simulink model "f4_variable_load"  (R2019b)
settings: Solver=VariableStepAuto  StartTime=0.0  StopTime=20  RelTol=1e-3
libraries: powerlib x28
settings Model: Creator=MAHMUD  LastModifiedBy=MAHMUD
settings DataIOCC: ReturnWorkspaceOutputs=off
settings DebuggingCC: ArithmeticOperatorsInVariantConditions=warning
settings SFSimCC: SimUseLocalCustomCode=off  CustomCodeUndefinedFunction=UseInterfaceOnly
settings RTWCC: RTWUseLocalCustomCode=off

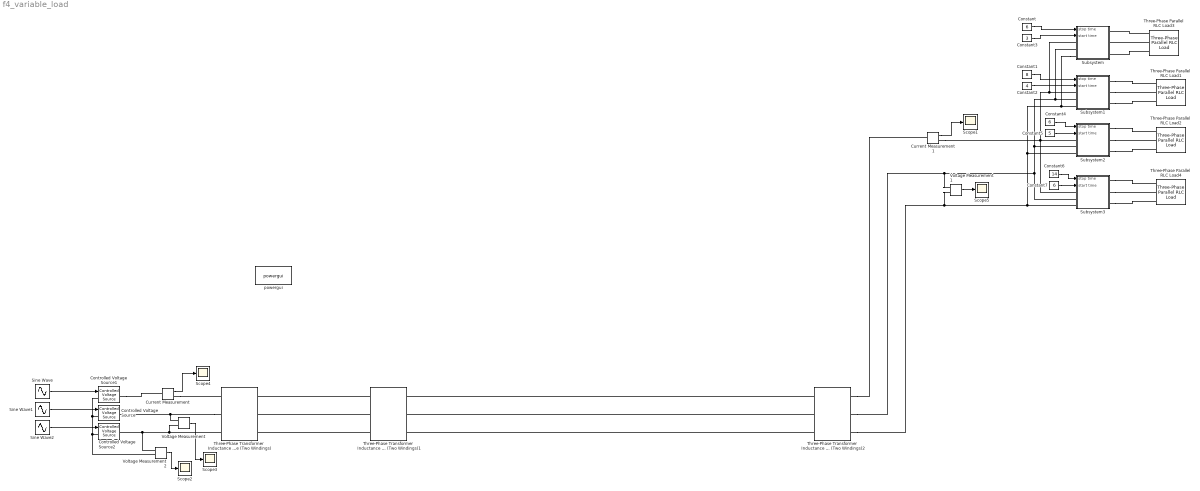
== system f4_variable_load ==
  Constant : Constant  Value=6
  Constant1 : Constant  Value=8
  Constant2 : Constant  Value=4
  Constant3 : Constant  Value=3
  Constant4 : Constant  Value=6
  Constant5 : Constant  Value=5
  Constant6 : Constant  Value=14
  Constant7 : Constant  Value=6
  Controlled Voltage Source : powerlib/Electrical Sources/Controlled Voltage Source  Initialize=on  Source_Type=AC  Amplitude=0  Phase=0  Frequency=0  Measurements=None
      settings: SourceProductName=Simscape Electrical
  Controlled Voltage Source1 : powerlib/Electrical Sources/Controlled Voltage Source  Initialize=on  Source_Type=AC  Amplitude=0  Phase=0  Frequency=0  Measurements=None
      settings: SourceProductName=Simscape Electrical
  Controlled Voltage Source2 : powerlib/Electrical Sources/Controlled Voltage Source  Initialize=on  Source_Type=AC  Amplitude=0  Phase=0  Frequency=0  Measurements=None
      settings: SourceProductName=Simscape Electrical
  Current Measurement : powerlib/Measurements/Current Measurement  PhasorSimulation=off  OutputType=Complex  PSBequivalent=0
      settings: SourceProductName=Simscape Electrical
  Current Measurement1 : powerlib/Measurements/Current Measurement  PhasorSimulation=off  OutputType=Complex  PSBequivalent=0
      settings: SourceProductName=Simscape Electrical
  Scope{1..5} (5 alike) : Scope
  Sine Wave : Sin  Amplitude=11500  Frequency=50*2*pi  SampleTime=0
  Sine Wave1 : Sin  Amplitude=11500  Frequency=50*2*pi  Phase=pi*2/3  SampleTime=0
  Sine Wave2 : Sin  Amplitude=11500  Frequency=50*2*pi  Phase=4*pi/3  SampleTime=0
  Subsystem : Subsystem
  Subsystem1 : Subsystem
  Subsystem2 : Subsystem
  Subsystem3 : Subsystem
  Three-Phase Parallel RLC Load1 : powerlib/Elements/Three-Phase Parallel RLC Load  LConnTagsString=A|B|C  Configuration=Y (grounded)  NominalVoltage=220  Vabc=[1e3 1e3 1e3]  Vabcp=[1e3 1e3 1e3]  NominalFrequency=50  UnbalancedPower=off  ActivePower=1.5e3  InductivePower=100  CapacitivePower=100  Pabc=[10e3 9e3 11e3]  QLabc=[100 90 110]  QCabc=[100 90 110]  Pabcp=[10e3 9e3 11e3]  QLabcp=[100 90 110]  QCabcp=[100 90 110]  Measurements=None  LoadType=constant Z
      settings: SourceProductName=Simscape Electrical
  Three-Phase Parallel RLC Load2 : powerlib/Elements/Three-Phase Parallel RLC Load  LConnTagsString=A|B|C  Configuration=Y (grounded)  NominalVoltage=220  Vabc=[1e3 1e3 1e3]  Vabcp=[1e3 1e3 1e3]  NominalFrequency=50  UnbalancedPower=off  ActivePower=1e3  InductivePower=100  CapacitivePower=100  Pabc=[10e3 9e3 11e3]  QLabc=[100 90 110]  QCabc=[100 90 110]  Pabcp=[10e3 9e3 11e3]  QLabcp=[100 90 110]  QCabcp=[100 90 110]  Measurements=None  LoadType=constant Z
      settings: SourceProductName=Simscape Electrical
  Three-Phase Parallel RLC Load3 : powerlib/Elements/Three-Phase Parallel RLC Load  LConnTagsString=A|B|C  Configuration=Y (grounded)  NominalVoltage=220  Vabc=[1e3 1e3 1e3]  Vabcp=[1e3 1e3 1e3]  NominalFrequency=50  UnbalancedPower=off  ActivePower=4e3  InductivePower=100  CapacitivePower=100  Pabc=[10e3 9e3 11e3]  QLabc=[100 90 110]  QCabc=[100 90 110]  Pabcp=[10e3 9e3 11e3]  QLabcp=[100 90 110]  QCabcp=[100 90 110]  Measurements=None  LoadType=constant Z
      settings: SourceProductName=Simscape Electrical
  Three-Phase Parallel RLC Load4 : powerlib/Elements/Three-Phase Parallel RLC Load  LConnTagsString=A|B|C  Configuration=Y (grounded)  NominalVoltage=220  Vabc=[1e3 1e3 1e3]  Vabcp=[1e3 1e3 1e3]  NominalFrequency=50  UnbalancedPower=off  ActivePower=12e3  InductivePower=100  CapacitivePower=100  Pabc=[10e3 9e3 11e3]  QLabc=[100 90 110]  QCabc=[100 90 110]  Pabcp=[10e3 9e3 11e3]  QLabcp=[100 90 110]  QCabcp=[100 90 110]  Measurements=None  LoadType=constant Z
      settings: SourceProductName=Simscape Electrical
  Three-Phase Transformer Inductance Matrix Type (Two Windings) : powerlib/Elements/Three-Phase Transformer Inductance Matrix Type (Two Windings)  CoreType=Three-limb or five-limb core  Winding1Connection=Yg  Winding2Connection=Yg  AutoTransformer=off  Measurements=None  NominalPower=[100e3, 50]  VLLnom=[25000, 130000]  WindingResistances=[0.01, 0.01]  NoLoadIexcPos=2  NoLoadPlossPos=1000  ShortCircuitReactancePos=0.06  ShortCircuitReactancePosAuto=0.06  NoLoadIexcZero=100  NoLoadPlossZero=1500  ShortCircuitReactanceZero=0.03  ShortCircuitReactanceZeroAuto=0.03
      settings: SourceProductName=Simscape Electrical  SourceProductBaseCode=PS
  Three-Phase Transformer Inductance Matrix Type (Two Windings)1 : powerlib/Elements/Three-Phase Transformer Inductance Matrix Type (Two Windings)  CoreType=Three-limb or five-limb core  Winding1Connection=Yg  Winding2Connection=Yg  AutoTransformer=off  Measurements=None  NominalPower=[100e3, 50]  VLLnom=[130000, 11000]  WindingResistances=[0.01, 0.01]  NoLoadIexcPos=2  NoLoadPlossPos=1000  ShortCircuitReactancePos=0.06  ShortCircuitReactancePosAuto=0.06  NoLoadIexcZero=100  NoLoadPlossZero=1500  ShortCircuitReactanceZero=0.03  ShortCircuitReactanceZeroAuto=0.03
      settings: SourceProductName=Simscape Electrical  SourceProductBaseCode=PS
  Three-Phase Transformer Inductance Matrix Type (Two Windings)2 : powerlib/Elements/Three-Phase Transformer Inductance Matrix Type (Two Windings)  CoreType=Three-limb or five-limb core  Winding1Connection=Yg  Winding2Connection=Yg  AutoTransformer=off  Measurements=None  NominalPower=[100e3, 50]  VLLnom=[11000, 381]  WindingResistances=[0.01, 0.01]  NoLoadIexcPos=2  NoLoadPlossPos=1000  ShortCircuitReactancePos=0.06  ShortCircuitReactancePosAuto=0.06  NoLoadIexcZero=100  NoLoadPlossZero=1500  ShortCircuitReactanceZero=0.03  ShortCircuitReactanceZeroAuto=0.03
      settings: SourceProductName=Simscape Electrical  SourceProductBaseCode=PS
  Voltage Measurement : powerlib/Measurements/Voltage Measurement  PhasorSimulation=off  OutputType=Complex  PSBequivalent=0
      settings: SourceProductName=Simscape Electrical
  Voltage Measurement1 : powerlib/Measurements/Voltage Measurement  PhasorSimulation=off  OutputType=Complex  PSBequivalent=0
      settings: SourceProductName=Simscape Electrical
  Voltage Measurement2 : powerlib/Measurements/Voltage Measurement  PhasorSimulation=off  OutputType=Complex  PSBequivalent=0
      settings: SourceProductName=Simscape Electrical
  powergui : powerlib/powergui  Priority=1  SimulationMode=Continuous  SampleTime=50e-6  frequency=60  Iterations=50  frequencyindice=50  Pbase=100e6  ErrMax=1e-4  UnitsV=kV  UnitsW=MW  buscounter=0  FunctionMessages=off  echomessages=off  EnableUseOfTLC=off  CurrentSourceSwitches=off  DisableSnubberDevices=off  DisableRonSwitches=off  DisableVfSwitches=off  DisplayEquations=off  AutomaticDiscreteSolvers=off  SolverType=Tustin/Backward Euler (TBE)  Interpol=off  ExternalGateDelay=off  methode=off  Ts=100  x0status=blocks  SPID=on  SwTol=0  HookPort=off  NonlinearTolerance=1e-4  nMaxIteration=100  ContinueOnMaxIteration=off  RestoreLinks=warning  ResistiveCurrentMeasurement=off  Frange=[0:2:500]  Ylog=off  Xlog=on  ShowGrid=off  save=off  variable=ZData  structure=0  ZoomFFT=off  StartTime=0.0  cycles=1  DisplayStyle=1  fundamental=60  FreqAxis=off  MaxFrequency=1000  frequencyindicesteady=1  RmsSteady=1  display=off
      settings: SourceProductName=Simscape Electrical
  wires:
  Voltage Measurement2/1 -> Scope2/1
  Constant5/1 -> Subsystem2/2(start time)
  Current Measurement/1 -> Scope4/1
  Constant1/1 -> Subsystem1/1(stop time)
  Constant6/1 -> Subsystem3/1(stop time)
  Sine Wave1/1 -> Controlled Voltage Source/1
  Sine Wave2/1 -> Controlled Voltage Source2/1
  Voltage Measurement1/1 -> Scope5/1
  Voltage Measurement/1 -> Scope3/1
  Constant7/1 -> Subsystem3/2(start time)
  Constant3/1 -> Subsystem/2(start time)
  Constant2/1 -> Subsystem1/2(start time)
  Constant/1 -> Subsystem/1(stop time)
  Constant4/1 -> Subsystem2/1(stop time)
  Sine Wave/1 -> Controlled Voltage Source1/1
  Current Measurement1/1 -> Scope1/1
  connections:
  Subsystem/LConn3 -- Subsystem1/LConn3 -- Subsystem2/LConn3 -- Voltage Measurement1/LConn2 -- Three-Phase Transformer Inductance Matrix Type (Two Windings)2/RConn3 -- Subsystem3/LConn3
  Controlled Voltage Source2/LConn1 -- Voltage Measurement2/LConn2 -- Controlled Voltage Source1/LConn1 -- Controlled Voltage Source/LConn1
  Three-Phase Transformer Inductance Matrix Type (Two Windings)/LConn2 -- Controlled Voltage Source/RConn1 -- Voltage Measurement/LConn1
  Three-Phase Transformer Inductance Matrix Type (Two Windings)2/RConn2 -- Voltage Measurement1/LConn1 -- Subsystem3/LConn2 -- Subsystem/LConn2 -- Subsystem1/LConn2 -- Subsystem2/LConn2
  Controlled Voltage Source2/RConn1 -- Voltage Measurement2/LConn1 -- Three-Phase Transformer Inductance Matrix Type (Two Windings)/LConn3 -- Voltage Measurement/LConn2
  Subsystem3/LConn1 -- Subsystem/LConn1 -- Subsystem1/LConn1 -- Subsystem2/LConn1 -- Current Measurement1/RConn1
  Three-Phase Transformer Inductance Matrix Type (Two Windings)2/LConn1 -- Three-Phase Transformer Inductance Matrix Type (Two Windings)1/RConn1
  Three-Phase Parallel RLC Load3/LConn2 -- Subsystem/RConn2
  Subsystem1/RConn2 -- Three-Phase Parallel RLC Load1/LConn2
  Three-Phase Parallel RLC Load3/LConn3 -- Subsystem/RConn3
  Three-Phase Transformer Inductance Matrix Type (Two Windings)2/LConn2 -- Three-Phase Transformer Inductance Matrix Type (Two Windings)1/RConn2
  Current Measurement/RConn1 -- Three-Phase Transformer Inductance Matrix Type (Two Windings)/LConn1
  Three-Phase Parallel RLC Load3/LConn1 -- Subsystem/RConn1
  Subsystem3/RConn3 -- Three-Phase Parallel RLC Load4/LConn3
  Controlled Voltage Source1/RConn1 -- Current Measurement/LConn1
  Three-Phase Transformer Inductance Matrix Type (Two Windings)2/LConn3 -- Three-Phase Transformer Inductance Matrix Type (Two Windings)1/RConn3
  Subsystem1/RConn3 -- Three-Phase Parallel RLC Load1/LConn3
  Three-Phase Transformer Inductance Matrix Type (Two Windings)1/LConn3 -- Three-Phase Transformer Inductance Matrix Type (Two Windings)/RConn3
  Three-Phase Transformer Inductance Matrix Type (Two Windings)2/RConn1 -- Current Measurement1/LConn1
  Subsystem3/RConn1 -- Three-Phase Parallel RLC Load4/LConn1
  Three-Phase Transformer Inductance Matrix Type (Two Windings)1/LConn2 -- Three-Phase Transformer Inductance Matrix Type (Two Windings)/RConn2
  Subsystem3/RConn2 -- Three-Phase Parallel RLC Load4/LConn2
  Subsystem1/RConn1 -- Three-Phase Parallel RLC Load1/LConn1
  Subsystem2/RConn1 -- Three-Phase Parallel RLC Load2/LConn1
  Three-Phase Transformer Inductance Matrix Type (Two Windings)1/LConn1 -- Three-Phase Transformer Inductance Matrix Type (Two Windings)/RConn1
  Subsystem2/RConn2 -- Three-Phase Parallel RLC Load2/LConn2
  Subsystem2/RConn3 -- Three-Phase Parallel RLC Load2/LConn3

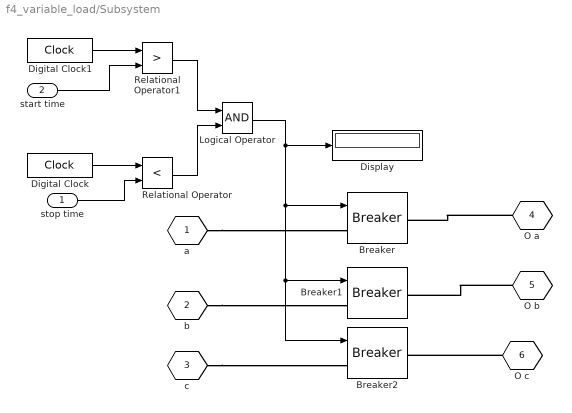
== system f4_variable_load/Subsystem ==
  stop time : Inport
  start time : Inport  Port=2
  Breaker : powerlib/Elements/Breaker  InitialState=0  SwitchingTimes="[1/60  5/60]"  External=on  BreakerResistance=0.01  SnubberResistance=1e6  SnubberCapacitance=inf  Measurements=None  MoreParameters=on  NoBreakLoop=off
      settings: SourceProductName=Simscape Electrical
  Breaker1 : powerlib/Elements/Breaker  InitialState=0  SwitchingTimes="[1/60  5/60]"  External=on  BreakerResistance=0.01  SnubberResistance=1e6  SnubberCapacitance=inf  Measurements=None  MoreParameters=on  NoBreakLoop=off
      settings: SourceProductName=Simscape Electrical
  Breaker2 : powerlib/Elements/Breaker  InitialState=0  SwitchingTimes="[1/60  5/60]"  External=on  BreakerResistance=0.01  SnubberResistance=1e6  SnubberCapacitance=inf  Measurements=None  MoreParameters=on  NoBreakLoop=off
      settings: SourceProductName=Simscape Electrical
  Digital Clock : DigitalClock
  Digital Clock1 : DigitalClock
  Display : Display
  Logical Operator : Logic  AllPortsSameDT=off  OutDataTypeStr=boolean
  Relational Operator : RelationalOperator  Operator=<  OutDataTypeStr=boolean  RndMeth=Simplest
  Relational Operator1 : RelationalOperator  Operator=>  OutDataTypeStr=boolean  RndMeth=Simplest
  a : PMIOPort  Tag=PMCPort  Side=Left
  b : PMIOPort  Tag=PMCPort  Port=2  Side=Left
  c : PMIOPort  Tag=PMCPort  Port=3  Side=Left
  "O a " : PMIOPort  Tag=PMCPort  Port=4  Side=Right
  O b : PMIOPort  Tag=PMCPort  Port=5  Side=Right
  O c : PMIOPort  Tag=PMCPort  Port=6  Side=Right
  wires:
  Logical Operator/1 -> Breaker/1, Breaker2/1, Breaker1/1, Display/1
  Digital Clock/1 -> Relational Operator/1
  stop time/1 -> Relational Operator/2
  Digital Clock1/1 -> Relational Operator1/1
  start time/1 -> Relational Operator1/2
  Relational Operator1/1 -> Logical Operator/1
  Relational Operator/1 -> Logical Operator/2
  connections:
  O c/RConn1 -- Breaker2/RConn1
  b/RConn1 -- Breaker1/LConn1
  O b/RConn1 -- Breaker1/RConn1
  c/RConn1 -- Breaker2/LConn1
  "O a "/RConn1 -- Breaker/RConn1
  a/RConn1 -- Breaker/LConn1

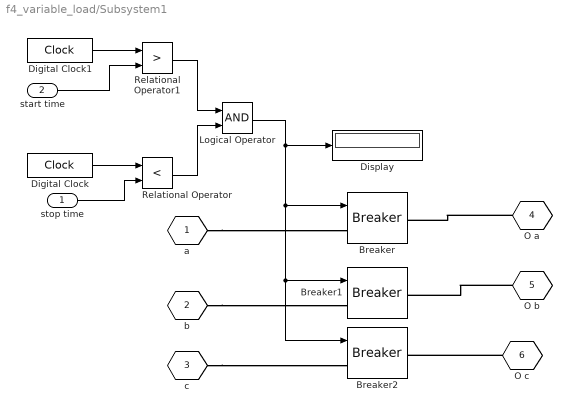
== system f4_variable_load/Subsystem1 ==
  stop time : Inport
  start time : Inport  Port=2
  Breaker : powerlib/Elements/Breaker  InitialState=0  SwitchingTimes="[1/60  5/60]"  External=on  BreakerResistance=0.01  SnubberResistance=1e6  SnubberCapacitance=inf  Measurements=None  MoreParameters=on  NoBreakLoop=off
      settings: SourceProductName=Simscape Electrical
  Breaker1 : powerlib/Elements/Breaker  InitialState=0  SwitchingTimes="[1/60  5/60]"  External=on  BreakerResistance=0.01  SnubberResistance=1e6  SnubberCapacitance=inf  Measurements=None  MoreParameters=on  NoBreakLoop=off
      settings: SourceProductName=Simscape Electrical
  Breaker2 : powerlib/Elements/Breaker  InitialState=0  SwitchingTimes="[1/60  5/60]"  External=on  BreakerResistance=0.01  SnubberResistance=1e6  SnubberCapacitance=inf  Measurements=None  MoreParameters=on  NoBreakLoop=off
      settings: SourceProductName=Simscape Electrical
  Digital Clock : DigitalClock
  Digital Clock1 : DigitalClock
  Display : Display
  Logical Operator : Logic  AllPortsSameDT=off  OutDataTypeStr=boolean
  Relational Operator : RelationalOperator  Operator=<  OutDataTypeStr=boolean  RndMeth=Simplest
  Relational Operator1 : RelationalOperator  Operator=>  OutDataTypeStr=boolean  RndMeth=Simplest
  a : PMIOPort  Tag=PMCPort  Side=Left
  b : PMIOPort  Tag=PMCPort  Port=2  Side=Left
  c : PMIOPort  Tag=PMCPort  Port=3  Side=Left
  "O a " : PMIOPort  Tag=PMCPort  Port=4  Side=Right
  O b : PMIOPort  Tag=PMCPort  Port=5  Side=Right
  O c : PMIOPort  Tag=PMCPort  Port=6  Side=Right
  wires:
  Relational Operator/1 -> Logical Operator/2
  Relational Operator1/1 -> Logical Operator/1
  start time/1 -> Relational Operator1/2
  Digital Clock1/1 -> Relational Operator1/1
  stop time/1 -> Relational Operator/2
  Digital Clock/1 -> Relational Operator/1
  Logical Operator/1 -> Display/1, Breaker1/1, Breaker2/1, Breaker/1
  connections:
  a/RConn1 -- Breaker/LConn1
  "O a "/RConn1 -- Breaker/RConn1
  c/RConn1 -- Breaker2/LConn1
  O b/RConn1 -- Breaker1/RConn1
  b/RConn1 -- Breaker1/LConn1
  O c/RConn1 -- Breaker2/RConn1

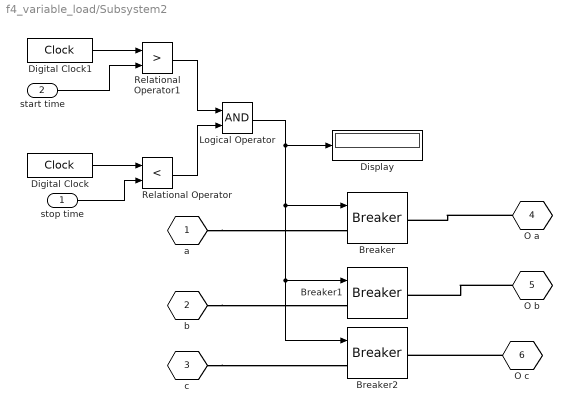
== system f4_variable_load/Subsystem2 ==
  stop time : Inport
  start time : Inport  Port=2
  Breaker : powerlib/Elements/Breaker  InitialState=0  SwitchingTimes="[1/60  5/60]"  External=on  BreakerResistance=0.01  SnubberResistance=1e6  SnubberCapacitance=inf  Measurements=None  MoreParameters=on  NoBreakLoop=off
      settings: SourceProductName=Simscape Electrical
  Breaker1 : powerlib/Elements/Breaker  InitialState=0  SwitchingTimes="[1/60  5/60]"  External=on  BreakerResistance=0.01  SnubberResistance=1e6  SnubberCapacitance=inf  Measurements=None  MoreParameters=on  NoBreakLoop=off
      settings: SourceProductName=Simscape Electrical
  Breaker2 : powerlib/Elements/Breaker  InitialState=0  SwitchingTimes="[1/60  5/60]"  External=on  BreakerResistance=0.01  SnubberResistance=1e6  SnubberCapacitance=inf  Measurements=None  MoreParameters=on  NoBreakLoop=off
      settings: SourceProductName=Simscape Electrical
  Digital Clock : DigitalClock
  Digital Clock1 : DigitalClock
  Display : Display
  Logical Operator : Logic  AllPortsSameDT=off  OutDataTypeStr=boolean
  Relational Operator : RelationalOperator  Operator=<  OutDataTypeStr=boolean  RndMeth=Simplest
  Relational Operator1 : RelationalOperator  Operator=>  OutDataTypeStr=boolean  RndMeth=Simplest
  a : PMIOPort  Tag=PMCPort  Side=Left
  b : PMIOPort  Tag=PMCPort  Port=2  Side=Left
  c : PMIOPort  Tag=PMCPort  Port=3  Side=Left
  "O a " : PMIOPort  Tag=PMCPort  Port=4  Side=Right
  O b : PMIOPort  Tag=PMCPort  Port=5  Side=Right
  O c : PMIOPort  Tag=PMCPort  Port=6  Side=Right
  wires:
  Logical Operator/1 -> Breaker/1, Breaker2/1, Breaker1/1, Display/1
  Digital Clock/1 -> Relational Operator/1
  stop time/1 -> Relational Operator/2
  Digital Clock1/1 -> Relational Operator1/1
  start time/1 -> Relational Operator1/2
  Relational Operator1/1 -> Logical Operator/1
  Relational Operator/1 -> Logical Operator/2
  connections:
  O c/RConn1 -- Breaker2/RConn1
  b/RConn1 -- Breaker1/LConn1
  O b/RConn1 -- Breaker1/RConn1
  c/RConn1 -- Breaker2/LConn1
  "O a "/RConn1 -- Breaker/RConn1
  a/RConn1 -- Breaker/LConn1

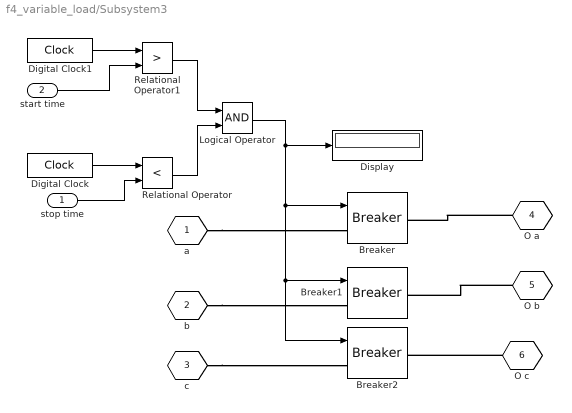
== system f4_variable_load/Subsystem3 ==
  stop time : Inport
  start time : Inport  Port=2
  Breaker : powerlib/Elements/Breaker  InitialState=0  SwitchingTimes="[1/60  5/60]"  External=on  BreakerResistance=0.01  SnubberResistance=1e6  SnubberCapacitance=inf  Measurements=None  MoreParameters=on  NoBreakLoop=off
      settings: SourceProductName=Simscape Electrical
  Breaker1 : powerlib/Elements/Breaker  InitialState=0  SwitchingTimes="[1/60  5/60]"  External=on  BreakerResistance=0.01  SnubberResistance=1e6  SnubberCapacitance=inf  Measurements=None  MoreParameters=on  NoBreakLoop=off
      settings: SourceProductName=Simscape Electrical
  Breaker2 : powerlib/Elements/Breaker  InitialState=0  SwitchingTimes="[1/60  5/60]"  External=on  BreakerResistance=0.01  SnubberResistance=1e6  SnubberCapacitance=inf  Measurements=None  MoreParameters=on  NoBreakLoop=off
      settings: SourceProductName=Simscape Electrical
  Digital Clock : DigitalClock
  Digital Clock1 : DigitalClock
  Display : Display
  Logical Operator : Logic  AllPortsSameDT=off  OutDataTypeStr=boolean
  Relational Operator : RelationalOperator  Operator=<  OutDataTypeStr=boolean  RndMeth=Simplest
  Relational Operator1 : RelationalOperator  Operator=>  OutDataTypeStr=boolean  RndMeth=Simplest
  a : PMIOPort  Tag=PMCPort  Side=Left
  b : PMIOPort  Tag=PMCPort  Port=2  Side=Left
  c : PMIOPort  Tag=PMCPort  Port=3  Side=Left
  "O a " : PMIOPort  Tag=PMCPort  Port=4  Side=Right
  O b : PMIOPort  Tag=PMCPort  Port=5  Side=Right
  O c : PMIOPort  Tag=PMCPort  Port=6  Side=Right
  wires:
  Relational Operator/1 -> Logical Operator/2
  Relational Operator1/1 -> Logical Operator/1
  start time/1 -> Relational Operator1/2
  Digital Clock1/1 -> Relational Operator1/1
  stop time/1 -> Relational Operator/2
  Digital Clock/1 -> Relational Operator/1
  Logical Operator/1 -> Display/1, Breaker1/1, Breaker2/1, Breaker/1
  connections:
  a/RConn1 -- Breaker/LConn1
  "O a "/RConn1 -- Breaker/RConn1
  c/RConn1 -- Breaker2/LConn1
  O b/RConn1 -- Breaker1/RConn1
  b/RConn1 -- Breaker1/LConn1
  O c/RConn1 -- Breaker2/RConn1
